simulink model "DcMotor"  (R2019a)
settings: Solver=VariableStepAuto  StartTime=0.0  StopTime=1  MaxStep=1e-3  RelTol=1e-3
settings Model: Creator=Roberto Strada  LastModifiedBy=Roberto Strada

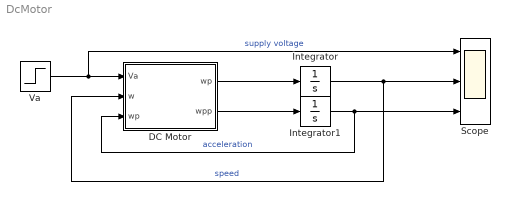
== system DcMotor ==
  DC Motor : MATLAB Function  TreatAsAtomicUnit=on
  Integrator : Integrator
  Integrator1 : Integrator
  Scope : Scope  NumInputPorts=3
  Va : Step  Time=0.1  After=10  SampleTime=0
  wires:
  Va/1 -> Scope/1, DC Motor/1(Va)  "supply voltage"
  DC Motor/1(wp) -> Integrator/1
  DC Motor/2(wpp) -> Integrator1/1
  Integrator1/1 -> Scope/3, DC Motor/3("wp ")  "acceleration"
  Integrator/1 -> DC Motor/2(w), Scope/2  "speed"

== matlab function DcMotor/DC Motor ==
  data: wp output; Va input; wpp output; w input; wp input
function [wp, wpp] = fcn(Va,w,wp)

Ra=3.3; La=20*3e-3; Jm=1.1e-4; K=0.122;
taue=La/Ra; taum=Ra*Jm/K^2;

wp=wp;
wpp = -wp/taue-w/(taue*taum)+Va/(K*taue*taum);
